simulink library "vmc"  (R2021b)
settings: Solver=VariableStepAuto  StartTime=0.0  StopTime=10.0  RelTol=1e-3
undefined symbols (not defined in the file): AVMC_ACCDeltaTqGradeGn_X_deg, AVMC_ACCDeltaTqIGain4OVRD_X_kph, AVMC_ACCDeltaTqIGain4OVRD_Y_mps2, AVMC_ACCDeltaTqIGain_X_kph, AVMC_ACCDeltaTqIGain_Y_mps2, AVMC_ACCDeltaTqPGain_X_kph, AVMC_ACCDeltaTqPGain_Y_kph, AVMC_ACCGradeofst_X_G, AVMC_ACCGradeofst_Y_pct, AVMC_ACCLoSpdTqLoLim4JP_X_kph, AVMC_ACCLoSpdTqLoLim4JP_Y_deg, AVMC_ACCLoSpdTqLowerLim_X_kph, AVMC_ACCLoSpdTqLowerLim_Y_deg, AVMC_ACCReqAccelGain_X_mps2, AVMC_ACCReqAccelGain_Y_enum, AVMC_ADSPosGFBDeltaTq_X_kph, AVMC_ADSPosGFBDeltaTq_Y_mps2, AVMC_AggressJerkPCT4AT_X_kph, AVMC_AggressJerkPCT_X_kph, AVMC_AggressLimitPCT4AT_X_kph, AVMC_AggressLimitPCT_X_kph, AVMC_DECGradeofst_X_G, AVMC_DECGradeofst_Y_pct, AVMC_DISCDeltaTqIGain_X_kph, AVMC_DISCDeltaTqIGain_Y_mps2, AVMC_DISCDeltaTqPGain_X_kph, AVMC_DISCDeltaTqPGain_Y_kph, AVMC_EPSForceSelect_X_enum, AVMC_EPSForceSelect_Y_enum, AVMC_EPSForceSelectD21_X_enum, AVMC_EPSForceSelectD21_Y_enum, AVMC_ESCRegenOut_X_kph, AVMC_ESCRegenOut_Y_Deg, AVMC_ESCRegenOutEnSpd_X_Deg, AVMC_EstPitchSlopeTs_X_kph, AVMC_GradeCompFlt_X_kph, AVMC_GyroYBandLo_X_Gps, AVMC_HoldResTq_X_kph, AVMC_ISOAccLimit_X_mps, AVMC_ISODecLimit_X_mps, AVMC_ISOJerk_X_mps, AVMC_LatESCRegenOut_X_kph, AVMC_LatESCRegenOut_Y_Deg, AVMC_LongAccDeadZone_X_kph, AVMC_LongAccFiltTsforP2_X_Gps, AVMC_MCPresBaseTq_X_bar, AVMC_MSAPedalOvrd_X_kph, AVMC_MSASpdBand_X_kph, AVMC_MSATqDownEndTq_X_kph, AVMC_MSATqDownTime_X_kph, AVMC_NegZCHoldTq_X_kph, AVMC_OPDDisSlideRate_X_Deg, AVMC_OVRD2ActSR2FCMCMD_X_mps2, AVMC_PedalTqRWhlRatio_X_Nm, AVMC_PedalTqRWhlRatio_Y_gps, AVMC_PedalTqRWhlSlipGain_X_rat, AVMC_PedalTqRWhlSlipGain_Y_kph, AVMC_PedalTqRWhSTRGGain_X_deg, AVMC_PedalTqRWhSTRGGain_Y_kph, AVMC_PosZCHoldTq_X_kph ... (+593)
libraries: hcu_lib x143, simulink x96, tqr x4, $bdroot x1, simulink_extras x1
(part 10 of 17)

== system vmc/VMC/VMC/IMU/IMU sensing result  ==
  VINP_SensingGyroX_raw16 : Inport
  VINP_SensingGyroY_raw16 : Inport  Port=2
  VINP_SensingGyroZ_raw16 : Inport  Port=3
  VINP_SensingAccX_raw16 : Inport  Port=4
  VINP_SensingAccY_raw16 : Inport  Port=5
  VINP_SensingAccZ_raw16 : Inport  Port=6
  VVMC_MemOffsetGyroX_Dps : Inport  Port=7
  VVMC_MemOffsetGyroY_Dps : Inport  Port=8
  VVMC_MemOffsetGyroZ_Dps : Inport  Port=9
  VVMC_MemOffsetAccX_G : Inport  Port=10
  VVMC_MemOffsetAccY_G : Inport  Port=11
  VVMC_MemOffsetAccZ_G : Inport  Port=12
  task_time_s : Inport  Port=13
  ACCEL_FS_SEL = 001 SENSITIVITY = 2000 LSB/g : Constant  Value=KVMC_AccFSSlect_enum
  Add{1..5,8} (6 alike) : Sum
  Cast To Single{1,4,7,10,14,17} (6 alike) : DataTypeConversion  OutDataTypeStr=single
  Cast To Single{2..3,5..6,8..9,11..13,15..16,18} (12 alike) : DataTypeConversion  OutDataTypeStr=uint8
  Constant{1..2,4,6} (4 alike) : Constant  Value=MINUSONE_FLOAT
  Constant{10,13,16,19..20,25} (6 alike) : Constant  Value=ZERO_FLOAT
  Constant{11,14,17,21..22,26,29..34} (12 alike) : Constant  Value=ONE_INT
  Constant12 : Constant  Value=KVMC_IMUGyroYRollAveLevel_enum
  Constant15 : Constant  Value=KVMC_IMUGyroZRollAveLevel_enum
  Constant18 : Constant  Value=KVMC_IMUAccXRollAveLevel_enum
  Constant23 : Constant  Value=KVMC_IMUGxFilter_raw32
  Constant24 : Constant  Value=KVMC_IMUAccYRollAveLevel_enum
  Constant27 : Constant  Value=KVMC_IMUGyroXRollAveLevel_enum
  Constant28 : Constant  Value=KVMC_IMUAccZRollAveLevel_enum
  Constant3 : Constant  Value=KVMC_IMURxFilter_raw32
  Constant5 : Constant  Value=KVMC_IMURzFilter_raw32
  Constant7 : Constant  Value=KVMC_IMUGzFilter_raw32
  Constant8 : Constant  Value=KVMC_IMUGyFilter_raw32
  Constant9 : Constant  Value=KVMC_IMURyFilter_raw32
  Data Type Conversion : DataTypeConversion  OutDataTypeStr=uint16
  Data Type Conversion{1..6} (6 alike) : DataTypeConversion  OutDataTypeStr=single
  Data Type Conversion7 : DataTypeConversion  OutDataTypeStr=uint16
  Divide{,1..9} (10 alike) : Product  Inputs=**
  FirstOrderFilter{1..6} (6 alike) : hcu_lib/Basic_Blocks/FirstOrderFilter
  GYRO_FS_SEL = 0001 SENSITIVITY = 50 LSB/dps : Constant  Value=KVMC_GyroFSSlect_enum
  Math Function{,1..5} (6 alike) : Math  Operator=reciprocal  SaturateOnIntegerOverflow=on
  Min{1..6} (6 alike) : MinMax  Function=max  Inputs=2
  Plus{,1..5} (6 alike) : Sum  Inputs=+-
  RollingAverage : Stateflow chart  TreatAsAtomicUnit=on
  RollingAverage1 : Stateflow chart  TreatAsAtomicUnit=on
  RollingAverage2 : Stateflow chart  TreatAsAtomicUnit=on
  RollingAverage3 : Stateflow chart  TreatAsAtomicUnit=on
  RollingAverage4 : Stateflow chart  TreatAsAtomicUnit=on
  RollingAverage5 : Stateflow chart  TreatAsAtomicUnit=on
  VVMC_CalibratedGyroX_Dps : Outport
  VVMC_CalibratedGyroY_Dps : Outport  Port=2
  VVMC_CalibratedGyroZ_Dps : Outport  Port=3
  VVMC_CalibratedAccX_G : Outport  Port=4
  VVMC_CalibratedAccY_G : Outport  Port=5
  VVMC_CalibratedAccZ_G : Outport  Port=6
  VVMC_CalibratedAccXAftRA_G : Outport  Port=7
  wires:
  [VVMC_CalibratedAccXAftRA_G] -> VVMC_CalibratedAccXAftRA_G/1
  Min6/1 -> RollingAverage5/1(KVMC_RollAveLevel_enum)
  Constant34/1 -> Min6/2
  Min5/1 -> RollingAverage4/1(KVMC_RollAveLevel_enum)
  Constant33/1 -> Min5/2
  Min4/1 -> RollingAverage3/1(KVMC_RollAveLevel_enum)
  Constant32/1 -> Min4/2
  Min2/1 -> RollingAverage2/1(KVMC_RollAveLevel_enum)
  Constant31/1 -> Min2/2
  Min1/1 -> RollingAverage1/1(KVMC_RollAveLevel_enum)
  Constant30/1 -> Min1/2
  Min3/1 -> RollingAverage/1(KVMC_RollAveLevel_enum)
  Constant29/1 -> Min3/2
  [VVMC_CalibratedAccZ_G] -> VVMC_CalibratedAccZ_G/1
  [VVMC_CalibratedAccY_G] -> VVMC_CalibratedAccY_G/1
  [VVMC_CalibratedAccX_G] -> VVMC_CalibratedAccX_G/1
  [VVMC_CalibratedGyroZ_Dps] -> VVMC_CalibratedGyroZ_Dps/1
  [VVMC_CalibratedGyroY_Dps] -> VVMC_CalibratedGyroY_Dps/1
  [VVMC_CalibratedGyroX_Dps] -> VVMC_CalibratedGyroX_Dps/1
  RollingAverage5/1(VVMC_RollAve_raw32) -> FirstOrderFilter3/1
  Constant25/1 -> Cast To Single17/1
  Constant28/1 -> Cast To Single16/1
  Cast To Single18/1 -> RollingAverage5/3(ONE_INT)
  Cast To Single16/1 -> Min6/1
  Cast To Single17/1 -> RollingAverage5/2(ZERO_FLOAT)
  Constant26/1 -> Cast To Single18/1
  RollingAverage4/1(VVMC_RollAve_raw32) -> FirstOrderFilter4/1
  Constant22/1 -> Cast To Single15/1
  Cast To Single14/1 -> RollingAverage4/2(ZERO_FLOAT)
  Cast To Single13/1 -> Min5/1
  Cast To Single15/1 -> RollingAverage4/3(ONE_INT)
  Constant24/1 -> Cast To Single13/1
  Constant19/1 -> Cast To Single14/1
  RollingAverage3/1(VVMC_RollAve_raw32) -> [VVMC_CalibratedAccXAftRA_G], FirstOrderFilter6/1  "VVMC_CalibratedAccXAftRA_G"
  Constant16/1 -> Cast To Single7/1
  Constant18/1 -> Cast To Single11/1
  Cast To Single8/1 -> RollingAverage3/3(ONE_INT)
  Cast To Single11/1 -> Min4/1
  Cast To Single7/1 -> RollingAverage3/2(ZERO_FLOAT)
  Constant17/1 -> Cast To Single8/1
  RollingAverage2/1(VVMC_RollAve_raw32) -> FirstOrderFilter2/1
  Cast To Single5/1 -> RollingAverage2/3(ONE_INT)
  Cast To Single4/1 -> RollingAverage2/2(ZERO_FLOAT)
  Cast To Single6/1 -> Min2/1
  Constant14/1 -> Cast To Single5/1
  Constant15/1 -> Cast To Single6/1
  Constant13/1 -> Cast To Single4/1
  RollingAverage1/1(VVMC_RollAve_raw32) -> FirstOrderFilter5/1
  Constant10/1 -> Cast To Single1/1
  Constant12/1 -> Cast To Single3/1
  Cast To Single2/1 -> RollingAverage1/3(ONE_INT)
  Cast To Single3/1 -> Min1/1
  Cast To Single1/1 -> RollingAverage1/2(ZERO_FLOAT)
  Constant11/1 -> Cast To Single2/1
  RollingAverage/1(VVMC_RollAve_raw32) -> FirstOrderFilter1/1
  Constant21/1 -> Cast To Single12/1
  Cast To Single10/1 -> RollingAverage/2(ZERO_FLOAT)
  Cast To Single9/1 -> Min3/1
  Cast To Single12/1 -> RollingAverage/3(ONE_INT)
  Constant27/1 -> Cast To Single9/1
  Constant20/1 -> Cast To Single10/1
  Plus1/1 -> RollingAverage1/4(VINP_INPData_raw32)
  Add5/1 -> FirstOrderFilter5/3
  Constant9/1 -> Add5/2
  [task_time_s] -> FirstOrderFilter5/2, Add5/1
  Plus4/1 -> RollingAverage4/4(VINP_INPData_raw32)
  [task_time_s] -> Add4/1, FirstOrderFilter4/2
  Constant8/1 -> Add4/2
  Add4/1 -> FirstOrderFilter4/3
  Plus5/1 -> Divide9/1
  [task_time_s] -> Add3/1, FirstOrderFilter3/2
  Constant7/1 -> Add3/2
  Add3/1 -> FirstOrderFilter3/3
  Constant6/1 -> Divide9/2
  Divide9/1 -> RollingAverage5/4(VINP_INPData_raw32)
  Plus2/1 -> Divide8/1
  Divide8/1 -> RollingAverage2/4(VINP_INPData_raw32)
  Constant4/1 -> Divide8/2
  Add2/1 -> FirstOrderFilter2/3
  Constant5/1 -> Add2/2
  [task_time_s] -> FirstOrderFilter2/2, Add2/1
  Plus/1 -> Divide7/1
  [task_time_s] -> Add1/1, FirstOrderFilter1/2
  Constant3/1 -> Add1/2
  Add1/1 -> FirstOrderFilter1/3
  Constant2/1 -> Divide7/2
  Divide7/1 -> RollingAverage/4(VINP_INPData_raw32)
  Divide6/1 -> RollingAverage3/4(VINP_INPData_raw32)
  Constant1/1 -> Divide6/2
  Add8/1 -> FirstOrderFilter6/3
  Constant23/1 -> Add8/2
  Plus3/1 -> Divide6/1
  [task_time_s] -> FirstOrderFilter6/2, Add8/1
  task_time_s/1 -> [task_time_s]
  Data Type Conversion6/1 -> Math Function5/1
  [VVMC_AccFSSlect_enum] -> Data Type Conversion6/1
  Data Type Conversion5/1 -> Math Function4/1
  Data Type Conversion4/1 -> Math Function3/1
  [VVMC_AccFSSlect_enum] -> Data Type Conversion4/1
  Data Type Conversion3/1 -> Math Function2/1
  Data Type Conversion2/1 -> Math Function1/1
  Data Type Conversion1/1 -> Math Function/1
  Math Function5/1 -> Divide5/2
  Math Function4/1 -> Divide4/2
  Math Function3/1 -> Divide3/2
  Math Function2/1 -> Divide2/2
  Math Function1/1 -> Divide1/2
  Math Function/1 -> Divide/2
  FirstOrderFilter3/1 -> [VVMC_CalibratedAccZ_G]  "VVMC_CalibratedAccZ_G"
  FirstOrderFilter4/1 -> [VVMC_CalibratedAccY_G]  "VVMC_CalibratedAccY_G"
  FirstOrderFilter6/1 -> [VVMC_CalibratedAccX_G]  "VVMC_CalibratedAccX_G"
  FirstOrderFilter2/1 -> [VVMC_CalibratedGyroZ_Dps]  "VVMC_CalibratedGyroZ_Dps"
  FirstOrderFilter5/1 -> [VVMC_CalibratedGyroY_Dps]  "VVMC_CalibratedGyroY_Dps"
  FirstOrderFilter1/1 -> [VVMC_CalibratedGyroX_Dps]  "VVMC_CalibratedGyroX_Dps"
  [VVMC_MemOffsetAccZ_G] -> Plus5/2
  [VVMC_SensingAccZ_G] -> Plus5/1
  [VVMC_MemOffsetAccY_G] -> Plus4/2
  [VVMC_SensingAccY_G] -> Plus4/1
  [VVMC_MemOffsetAccX_G] -> Plus3/2
  [VVMC_SensingAccX_G] -> Plus3/1
  [VVMC_MemOffsetGyroZ_Dps] -> Plus2/2
  [VVMC_SensingGyroZ_Dps] -> Plus2/1
  [VVMC_MemOffsetGyroY_Dps] -> Plus1/2
  [VVMC_SensingGyroY_Dps] -> Plus1/1
  [VVMC_MemOffsetGyroX_Dps] -> Plus/2
  [VVMC_SensingGyroX_Dps] -> Plus/1
  Divide/1 -> [VVMC_SensingGyroX_Dps]  "VVMC_SensingGyroX_Dps"
  Divide5/1 -> [VVMC_SensingAccZ_G]  "VVMC_SensingAccZ_G"
  VINP_SensingAccZ_raw16/1 -> [VINP_SensingAccZ_raw16]
  VINP_SensingAccY_raw16/1 -> [VINP_SensingAccY_raw16]
  VINP_SensingAccX_raw16/1 -> [VINP_SensingAccX_raw16]
  VINP_SensingGyroZ_raw16/1 -> [VINP_SensingGyroZ_raw16]
  VINP_SensingGyroY_raw16/1 -> [VINP_SensingGyroY_raw16]
  VINP_SensingGyroX_raw16/1 -> [VINP_SensingGyroX_raw16]
  VVMC_MemOffsetAccX_G/1 -> [VVMC_MemOffsetAccX_G]
  VVMC_MemOffsetGyroZ_Dps/1 -> [VVMC_MemOffsetGyroZ_Dps]
  VVMC_MemOffsetAccZ_G/1 -> [VVMC_MemOffsetAccZ_G]
  VVMC_MemOffsetAccY_G/1 -> [VVMC_MemOffsetAccY_G]
  VVMC_MemOffsetGyroX_Dps/1 -> [VVMC_MemOffsetGyroX_Dps]
  VVMC_MemOffsetGyroY_Dps/1 -> [VVMC_MemOffsetGyroY_Dps]
  [VINP_SensingGyroX_raw16] -> Divide/1
  [VVMC_GyroFSSlect_enum] -> Data Type Conversion1/1
  GYRO_FS_SEL = 0001 SENSITIVITY = 50 LSB/dps/1 -> Data Type Conversion/1
  Data Type Conversion/1 -> [VVMC_GyroFSSlect_enum]  "VVMC_GyroFSSlect_enum"
  [VVMC_GyroFSSlect_enum] -> Data Type Conversion2/1
  [VINP_SensingGyroY_raw16] -> Divide1/1
  [VINP_SensingGyroZ_raw16] -> Divide2/1
  [VVMC_GyroFSSlect_enum] -> Data Type Conversion3/1
  [VINP_SensingAccX_raw16] -> Divide3/1
  [VINP_SensingAccY_raw16] -> Divide4/1
  [VVMC_AccFSSlect_enum] -> Data Type Conversion5/1
  [VINP_SensingAccZ_raw16] -> Divide5/1
  Data Type Conversion7/1 -> [VVMC_AccFSSlect_enum]  "VVMC_AccFSSlect_enum"
  ACCEL_FS_SEL = 001 SENSITIVITY = 2000 LSB/g/1 -> Data Type Conversion7/1
  Divide1/1 -> [VVMC_SensingGyroY_Dps]  "VVMC_SensingGyroY_Dps"
  Divide2/1 -> [VVMC_SensingGyroZ_Dps]  "VVMC_SensingGyroZ_Dps"
  Divide3/1 -> [VVMC_SensingAccX_G]  "VVMC_SensingAccX_G"
  Divide4/1 -> [VVMC_SensingAccY_G]  "VVMC_SensingAccY_G"

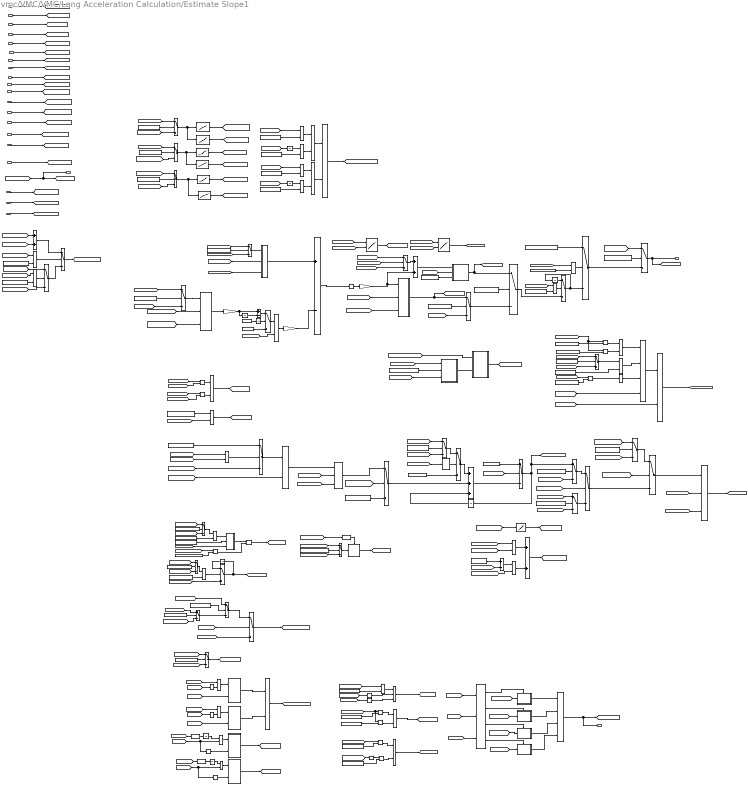
== system vmc/VMC/VMC/Long Acceleration Calculation/Estimate Slope1 ==
  VINP_LongAccel_Gps : Inport
  VINP_VehSpeed_kph : Inport  Port=2
  VINP_GRADE_deg : Inport  Port=3
  VVMC_CalibratedGyroY_Dps : Inport  Port=4
  VVMC_CalibratedAccX_G : Inport  Port=5
  VVMC_CalibratedAccY_G : Inport  Port=6
  VVMC_CalibratedAccZ_G : Inport  Port=7
  C_TASK_10MS_S : Inport  Port=8
  VDHP_ActAPSPosn_pct : Inport  Port=9
  VTQD_GearActualPosn_enum : Inport  Port=10
  VTQD_PreLoadPreEn_flg : Inport  Port=11
  VINP_BrkPedalPos_pct : Inport  Port=12
  VTQD_VehActSpd_kph : Inport  Port=13
  VTQD_RegenMode_enum : Inport  Port=14
  VINP_DIDGetDynoMode_flg : Inport  Port=15
  VVMC_HoldEstSlope_deg : Inport  Port=16
  VVMC_InitEstSlope_Deg : Inport  Port=17
  VTQR_RrTMTqReq_Nm : Inport  Port=18
  VTQR_FrTMTqReq_Nm : Inport  Port=19
  VPMM_DrivetrainSelect_enum : Inport  Port=20
  AND{,2..12} (12 alike) : Logic  AllPortsSameDT=off  OutDataTypeStr=boolean
  AND1 : Logic  Inputs=4  AllPortsSameDT=off  OutDataTypeStr=boolean
  AND13 : Logic  Inputs=3  AllPortsSameDT=off  OutDataTypeStr=boolean
  Abs : Abs
  Add : Sum
  Add1 : Sum  Inputs=+-
  Add2 : Sum  Inputs=+++
  Add3 : Sum
  Add5 : Sum
  Asin1 : Trigonometry  Operator=asin
  Constant : Constant  Value=KVMC_EstSlopeVehSourceSW_flg
  Constant1 : Constant  Value=KVMC_VehRunSlope_flg
  Constant{10,12,25,31,53} (5 alike) : Constant  Value=ZERO_FLOAT
  Constant11 : Constant  Value=KVMC_PitchVehThres_kph
  Constant13 : Constant  Value=KVMC_VehStopAPSThresLo_pct
  Constant14 : Constant  Value=KVMC_DIDGetDynoModeSW_flg
  Constant{15,36,50..51} (4 alike) : Constant  Value=KVMC_SlopeCalSource_flg
  Constant16 : Constant  Value=KVMC_PitchBPSThres_pct
  Constant17 : Constant  Value=ENUM_GEARSHIFTCMD_D
  Constant18 : Constant  Value=ENUM_GEARSHIFTCMD_R
  Constant19 : Constant  Value=ENUM_GEARSHIFTCMD_R
  Constant2 : Constant  Value=ENUM_DRIVETRAIN_AWD
  Constant20 : Constant  Value=KVMC_GyroBandSource_flg
  Constant21 : Constant  Value=ENUM_GEARSHIFTCMD_D
  Constant22 : Constant  Value=KVMC_GradedelayTimer_s
  Constant23 : Constant  Value=KVMC_VehStopSource_flg
  Constant24 : Constant  Value=KVMC_GradedelaytestSW_flg
  Constant26 : Constant  Value=KVMC_PitchGradeReset_flg
  Constant27 : Constant  Value=KVMC_PitchGradeStopSource_flg
  Constant29 : Constant  Value=KVMC_PitchGradeStopSource_flg
  Constant3 : Constant  Value=ENUM_DRIVETRAIN_RWD
  Constant30 : Constant  Value=KVMC_VehStopThres_kph
  Constant32 : Constant  Value=KVMC_VehStopDelay_s
  Constant33 : Constant  Value=KVMC_VehStopThresLo_kph
  Constant34 : Constant  Value=KVMC_VehStopThresHi_kph
  Constant35 : Constant  Value=KVMC_VehStopThresHi_kph
  Constant38 : Constant  Value=KVMC_VehStopThresLo_kph
  Constant39 : Constant  Value=KVMC_EstSlopeVehSourceSW_flg
  Constant4 : Constant  Value=KVMC_VehStopTqThres_Nm
  Constant42 : Constant  Value=KVMC_EstSlopeSW_flg
  Constant47 : Constant  Value=KVMC_CalEstSlopeOfst_c
  Constant48 : Constant  Value=KVMC_CalEstSlopeOfstSW_flg
  Constant49 : Constant  Value=KVMC_FreezeStopGrade_kph
  Constant5 : Constant  Value=ONE_FLOAT
  Constant52 : Constant  Value=KVMC_EstSlopeLongGSW_flg
  Constant54 : Constant  Value=KVMC_PitchAccGup_mps2
  Constant55 : Constant  Value=KVMC_PitchAccGlow_mps2
  Constant56 : Constant  Value=KVMC_EstSlopeVehSourceSW_flg
  Constant57 : Constant  Value=KVMC_StoploopGradeSource_flg
  Constant6 : Constant  Value=KVMC_PitchGradeL2HSource_flg
  Constant60 : Constant  Tag=struct('comment',struct('text','','placement',1),'output',struct('width',1,'name','$S_$B','unit','','type','Int16','offset',0,'max',NaN,'min',NaN,'freeze',1,'lsb',1,'arb',0,'class','default','address','','description','','value','2','tolerance',1,'show',0),'date',731450.690075)  Value=TRUE
  Constant7 : Constant  Value=KVMC_VehStopSource_flg
  Constant8 : Constant  Tag=struct('comment',struct('text','','placement',1),'output',struct('width',1,'name','$S_$B','unit','','type','Int16','offset',0,'max',NaN,'min',NaN,'freeze',1,'lsb',1,'arb',0,'class','default','address','','description','','value','0','tolerance',1,'show',0),'date',731450.689904282)  Value=ZERO_FLOAT  OutDataTypeStr=single
  Constant9 : Constant  Value=KVMC_SlopeSourceTs_flg
  DelayEnable : Subsystem  mask(DelayEnable){}
      mask help: Delay enable funcion.
  DelayEnable4 : Subsystem  mask(DelayEnable){}
      mask help: Delay enable funcion.
  Detect Decrease{,1..3} (4 alike) : simulink/Logic and Bit Operations/Detect Decrease  vinit=0.0  OutDataTypeStr=boolean
  Equal{,1..5} (6 alike) : RelationalOperator  Operator===  OutDataTypeStr=boolean  RndMeth=Simplest
  FirstOrderFilter3 : Subsystem  RTWFileName=HCU_LIB  mask(FirstOrderFilter){}
      mask help: First order Filter.
      settings: RTWFileNameOpts=User specified
  FirstOrderFilter4 : Subsystem  RTWFileName=HCU_LIB  mask(FirstOrderFilter){}
      mask help: First order Filter.
      settings: RTWFileNameOpts=User specified
  FirstOrderFilter5 : Subsystem  RTWFileName=HCU_LIB  mask(FirstOrderFilter){}
      mask help: First order Filter.
      settings: RTWFileNameOpts=User specified
  FirstOrderFilter6 : Subsystem  RTWFileName=HCU_LIB  mask(FirstOrderFilter){}
      mask help: First order Filter.
      settings: RTWFileNameOpts=User specified
  FirstOrderFilter7 : Subsystem  RTWFileName=HCU_LIB  mask(FirstOrderFilter){}
      mask help: First order Filter.
      settings: RTWFileNameOpts=User specified
  FirstOrderFilter8 : Subsystem  RTWFileName=HCU_LIB  mask(FirstOrderFilter){}
      mask help: First order Filter.
      settings: RTWFileNameOpts=User specified
  Gain : Gain  Gain=KPH2MPS
  Gain1 : Gain  Gain=1/GRAVITY_G
  Gain5 : Gain  Gain=RAD2DEG
  GreaterThan : RelationalOperator  Operator=<  OutDataTypeStr=boolean  RndMeth=Simplest
  GreaterThan2 : RelationalOperator  OutDataTypeStr=boolean  RndMeth=Simplest
  GreaterThan3 : RelationalOperator  Operator=>  OutDataTypeStr=boolean  RndMeth=Simplest
  GreaterThan4 : RelationalOperator  Operator=>  OutDataTypeStr=boolean  RndMeth=Simplest
  GreaterThan5 : RelationalOperator  Operator=>  OutDataTypeStr=boolean  RndMeth=Simplest
  If : If  NumInputs=3  IfExpression=u1 ~= 0  ElseIfExpressions=u2 ~= 0, u3~=0
  If Action Subsystem : Subsystem  TreatAsAtomicUnit=on
  If Action Subsystem1 : Subsystem  TreatAsAtomicUnit=on
  If Action Subsystem2 : Subsystem  TreatAsAtomicUnit=on
  If Action Subsystem3 : Subsystem  TreatAsAtomicUnit=on
  Less Than : RelationalOperator  Operator=>  OutDataTypeStr=boolean  RndMeth=Simplest
  Less Than{1..2,5..8} (6 alike) : RelationalOperator  Operator=<  OutDataTypeStr=boolean  RndMeth=Simplest
  Less Than3 : RelationalOperator  OutDataTypeStr=boolean  RndMeth=Simplest
  Less Than4 : RelationalOperator  Operator=<=  OutDataTypeStr=boolean  RndMeth=Simplest
  MVMC_ACCGradeofst_Deg : Lookup_n-D  BreakpointsForDimension1=AVMC_ACCGradeofst_Y_pct  BreakpointsForDimension2=AVMC_ACCGradeofst_X_G  Table=MVMC_ACCGradeofst_Z_Deg  InternalRulePriority=Speed  RndMeth=Simplest  InputSameDT=on
      settings: InputPortMap=u0,u1
  MVMC_CalEstSlopeTs_Y_c : Lookup_n-D  NumberOfTableDimensions=1  BreakpointsForDimension1=AVMC_EstPitchSlopeTs_X_kph  Table=MVMC_CalEstSlopeTs_Y_c  InternalRulePriority=Speed  RndMeth=Simplest  InputSameDT=on
  MVMC_CalibratedGyroYDevTs_Y_c : Lookup_n-D  NumberOfTableDimensions=1  BreakpointsForDimension1=AVMC_EstPitchSlopeTs_X_kph  Table=MVMC_CalibratedGyroYDevTs_Y_c  InternalRulePriority=Speed  RndMeth=Simplest  InputSameDT=on
  MVMC_DECGradeofst_Deg : Lookup_n-D  BreakpointsForDimension1=AVMC_DECGradeofst_Y_pct  BreakpointsForDimension2=AVMC_DECGradeofst_X_G  Table=MVMC_DECGradeofst_Z_Deg  InternalRulePriority=Speed  RndMeth=Simplest  InputSameDT=on
      settings: InputPortMap=u0,u1
  MVMC_EstPitchSlopeTs_Y_c : Lookup_n-D  NumberOfTableDimensions=1  BreakpointsForDimension1=AVMC_EstPitchSlopeTs_X_kph  Table=MVMC_EstPitchSlopeTs_Y_c  InternalRulePriority=Speed  RndMeth=Simplest  InputSameDT=on
  MVMC_GradeCompFlt_Y_c : Lookup_n-D  NumberOfTableDimensions=1  BreakpointsForDimension1=AVMC_GradeCompFlt_X_kph  Table=MVMC_GradeCompFlt_Y_c  InternalRulePriority=Speed  RndMeth=Simplest  InputSameDT=on
  MVMC_GyroYBandHi_Y_Dps : Lookup_n-D  NumberOfTableDimensions=1  BreakpointsForDimension1=AVMC_GyroYBandLo_X_Gps  Table=MVMC_GyroYBandHi_Y_Dps  InternalRulePriority=Speed  RndMeth=Simplest  InputSameDT=on
  MVMC_GyroYBandLo_Y_Dps : Lookup_n-D  NumberOfTableDimensions=1  BreakpointsForDimension1=AVMC_GyroYBandLo_X_Gps  Table=MVMC_GyroYBandLo_Y_Dps  InternalRulePriority=Speed  RndMeth=Simplest  InputSameDT=on
  MVMC_VehspdTs_Y_c : Lookup_n-D  NumberOfTableDimensions=1  BreakpointsForDimension1=AVMC_EstPitchSlopeTs_X_kph  Table=MVMC_VehspdTs_Y_c  InternalRulePriority=Speed  RndMeth=Simplest  InputSameDT=on
  Merge : Merge  Inputs=4
  NOT{,1..4,7..8} (7 alike) : Logic  Operator=NOT  AllPortsSameDT=off  OutDataTypeStr=boolean
  OR{,3,5..7} (5 alike) : Logic  Operator=OR  AllPortsSameDT=off  OutDataTypeStr=boolean
  OR1 : Logic  AllPortsSameDT=off  OutDataTypeStr=boolean
  Product : Product
  Product1 : Product
  Product2 : Product
  Product4 : Product  Tag=struct('comment',struct('text','','placement',1),'logdata',struct('maxnumvals',inf,'plotchannels',[],'stepsize',0,'downsampling',1,'loggingmode',3,'channels',1),'output',struct('width',1,'name','$S_$B','unit','','type','Int32Bin15','offset',0,'max',65535,'min',-65536,'freeze',1,'lsb',2^-15,'arb',0,'class','default','address','','description','','autoscalingmode',1,'lowerheadroom',1,'upperheadroom',1,'headroomunit','bit','checkmin',0,'checkmax',0,'show',0),'inputs','*/','exceptionhandling',1,'date',731458.438505301)  Inputs=*/  InputSameDT=on  RndMeth=Zero  SaturateOnIntegerOverflow=on  OutDataTypeStr=Inherit: Same as first input
  SR_Latch : Subsystem  mask(SR_Latch){}
      mask help: SR latch function.
  SR_Latch1 : Subsystem  mask(SR_Latch){}
      mask help: SR latch function.
  SR_Latch2 : Subsystem  mask(SR_Latch){}
      mask help: SR latch function.
  SR_Latch3 : Subsystem  mask(SR_Latch){}
      mask help: SR latch function.
  SR_Latch6 : Subsystem  mask(SR_Latch){}
      mask help: SR latch function.
  Subtract : Sum  Inputs=+-
  Sum1 : Sum  Tag=struct('comment',struct('text','','placement',1),'logdata',struct('maxnumvals',inf,'plotchannels',[],'stepsize',0,'downsampling',1,'loggingmode',3,'channels',1),'output',struct('width',1,'name','$S_$B','unit','','type','Int32Bin15','offset',0,'max',65535,'min',-65536,'freeze',1,'lsb',2^-15,'arb',0,'class','default','address','','description','','autoscalingmode',1,'lowerheadroom',1,'upperheadroom',1,'headroomunit','bit','checkmin',0,'checkmax',0,'show',0),'inputs','+-','date',731450.688943275)  Inputs=+-  InputSameDT=on  SaturateOnIntegerOverflow=on  OutDataTypeStr=Inherit: Same as first input
  Switch{,1..3,8,12,14..23,25..28,30..31,33} (23 alike) : Switch  Criteria=u2 > Threshold
  Switch{4..7,9..11,32} (8 alike) : Switch  Criteria=u2 ~= 0
  Switch13 : Switch
  Switch35 : Switch  Tag=struct('comment',struct('text','','placement',1),'logdata',struct('maxnumvals',inf,'plotchannels',[],'stepsize',0,'downsampling',1,'loggingmode',3,'channels',1),'output',struct('width',1,'name','$S_$B','unit','','type','Int32Bin15','offset',0,'max',65535,'min',-65536,'freeze',1,'lsb',2^-15,'arb',0,'class','default','address','','description','','autoscalingmode',1,'lowerheadroom',1,'upperheadroom',1,'headroomunit','bit','checkmin',0,'checkmax',0,'show',0),'threshold',struct('width',1,'name','$S_$B_threshold','unit','','type','Int16','offset',0,'max',NaN,'min',NaN,'freeze',1,'lsb',1,'arb',0,'class','default','address','','description','','value','1','scalar',0),'date',731458.438569977)  Criteria=u2 > Threshold  SaturateOnIntegerOverflow=on  InputSameDT=on
  Triggered Subsystem : Subsystem  TreatAsAtomicUnit=on
  Unit Delay{,1..5,8} (7 alike) : UnitDelay  SampleTime=-1  HasFrameUpgradeWarning=on
  UnitDelay3 : UnitDelay  Tag=struct('comment',struct('text','','placement',1),'logdata',struct('maxnumvals',inf,'plotchannels',[],'stepsize',0,'downsampling',1,'loggingmode',3,'channels',1),'output',struct('width',1,'name','$S_$B','unit','','type','Int32Bin15','offset',0,'max',65535,'min',-65536,'freeze',1,'lsb',2^-15,'arb',0,'class','default','address','','description','','autoscalingmode',1,'lowerheadroom',1,'upperheadroom',1,'headroomunit','bit','checkmin',0,'checkmax',0,'show',0,'initial','0'),'state',0,'dt','-1','date',731450.687911019)  SampleTime=-1  HasFrameUpgradeWarning=on
  UnitDelay4 : UnitDelay  Tag=struct('comment',struct('text','','placement',1),'logdata',struct('maxnumvals',inf,'plotchannels',[],'stepsize',0,'downsampling',1,'loggingmode',3,'channels',1),'output',struct('width',1,'name','$S_$B','unit','','type','UInt8','offset',0,'max',255,'min',0,'freeze',1,'lsb',1,'arb',0,'class','default','address','','description','','autoscalingmode',1,'lowerheadroom',1,'upperheadroom',1,'headroomunit','bit','checkmin',0,'checkmax',0,'show',0,'initial','0'),'state',0,'dt','-1','date',731450.690382801)  InitialCondition=FALSE  SampleTime=-1  StateName=first_pass  HasFrameUpgradeWarning=on
  VVMC_EstSlopeCalBase_Deg : Outport
  VVMC_IMUEstSlope_Deg1 : Outport  Port=2
  VVMC_FinalSlop_deg : Outport  Port=3
  wires:
  C_TASK_10MS_S/1 -> [task_time_s]
  [VINP_GRADE_deg] -> Switch1/3
  [VINP_LongAccel_Gps] -> Switch3/3
  VVMC_CalibratedAccZ_G/1 -> [VVMC_CalibratedAccZ_G]
  VVMC_CalibratedAccY_G/1 -> [VVMC_CalibratedAccY_G]
  Switch33/1 -> Switch26/1
  [VVMC_PitchIntegGradeMen_deg] -> Switch33/1
  Constant57/1 -> Switch33/2
  [VVMC_PitchIntegGradeMen_deg] -> Switch26/3
  [VVMC_EstSlopeCalBase_Deg] -> Switch/1
  [VVMC_DECGradeofst_Deg] -> Switch22/3
  FirstOrderFilter4/1(out) -> Gain/1
  SR_Latch6/1(latched) -> [VVMC_GradeShiftDelay_flg]  "VVMC_GradeShiftDelay_flg"
  [VVMC_EstSlopeCalBase_Deg] -> Switch30/1
  [VVMC_StopGrade_deg] -> If Action Subsystem2/1(In1)
  Constant17/1 -> Equal2/2
  Switch30/1 -> Switch13/1
  Switch4/1 -> FirstOrderFilter4/1(in)
  [VINP_BrkPedalPos_pct] -> MVMC_DECGradeofst_Deg/1
  [VVMC_EstSlopeCalBase_Deg] -> Switch31/1
  GreaterThan3/1 -> NOT/1
  MVMC_GyroYBandHi_Y_Dps/1 -> [VVMC_GyroYBandHigh_Dps]  "VVMC_GyroYBandHigh_Dps"
  AND10/1 -> SR_Latch2/1(set)
  [VVMC_GyroYBand_flg] -> OR3/1
  [VTQD_VehActSpd_kph] -> Switch4/1
  Switch2/1 -> Switch31/3
  [task_time_s] -> FirstOrderFilter4/2(Tc)
  DelayEnable/1(set) -> AND9/1
  [VVMC_EstSlopeCalBase_Deg] -> Switch28/1
  FirstOrderFilter5/1(out) -> Switch1/1, [VVMC_CalEstSlope1_Deg]  "VVMC_CalEstSlope1_Deg"
  [task_time_s] -> FirstOrderFilter6/2(Tc)
  [VTQD_PreLoadPreEn_flg] -> DelayEnable4/1(trigger)
  [VDHP_ActAPSPosn_pct] -> MVMC_ACCGradeofst_Deg/1
  [VVMC_CalibratedGyroY_Dps] -> GreaterThan4/1
  Constant26/1 -> OR7/1
  [VVMC_ACCGradeofst_Deg] -> Switch22/1
  [VTQD_VehActSpd_kph] -> Switch20/1
  Less Than1/1 -> OR1/2
  [VVMC_GradeReset_flg] -> Switch12/2
  [VVMC_CalibratedAccX_G] -> MVMC_DECGradeofst_Deg/2
  Switch22/1 -> Add5/1
  [VVMC_Vehfullstop_flg] -> Switch26/2
  FirstOrderFilter8/1(out) -> [VVMC_CalEstSlopeOfstA_Deg], Switch23/1  "VVMC_CalEstSlopeOfstA_Deg"
  MVMC_CalibratedGyroYDevTs_Y_c/1 -> [VVMC_CalibratedGyroYDevTs_c]  "VVMC_CalibratedGyroYDevTs_c"
  [VVMC_CalibratedAccX_G] -> Switch10/1
  Merge/1 -> [VVMC_FinalSlop_deg], VVMC_FinalSlop_deg/1  "VVMC_FinalSlop_deg"
  Switch9/1 -> Product/1
  [VVMC_HoldEstSlope_deg] -> Switch28/3
  [VVMC_GyroYBandLow_Dps] -> GreaterThan4/2
  Switch15/1 -> MVMC_VehspdTs_Y_c/1, MVMC_CalEstSlopeTs_Y_c/1
  Constant39/1 -> Switch32/2
  If Action Subsystem2/1(Out1) -> Merge/3
  Constant32/1 -> DelayEnable/2(T_delay)
  Constant53/1 -> Switch2/1
  [VINP_VehSpeed_kph] -> Switch20/3
  Constant47/1 -> FirstOrderFilter8/3(Ts)
  Add5/1 -> FirstOrderFilter8/1(in)  "VVMC_CalEstSlopeOfstB_Deg"
  Constant21/1 -> Equal4/2
  Constant9/1 -> Switch15/2
  Switch16/1 -> Triggered Subsystem/1(In1)
  [task_time_s] -> FirstOrderFilter3/2(Tc)
  [VTQD_VehActSpd_kph] -> Switch15/3
  Constant54/1 -> GreaterThan/2
  [VVMC_CalibratedAccX_G] -> Switch15/1
  If/1 -> If Action Subsystem/Action
  MVMC_DECGradeofst_Deg/1 -> [VVMC_DECGradeofst_Deg]  "VVMC_DECGradeofst_Deg"
  [VVMC_GyroYBandHigh_Dps] -> Less Than1/2
  MVMC_ACCGradeofst_Deg/1 -> [VVMC_ACCGradeofst_Deg]  "VVMC_ACCGradeofst_Deg"
  Constant34/1 -> Less Than4/2
  Gain5/1 -> FirstOrderFilter5/1(in), Add5/2  "VVMC_CalEstSlopeBefore_Deg"
  OR1/1 -> [VVMC_GyroYBand_flg]  "VVMC_GyroYBand_flg"
  [VVMC_GradeReset_flg] -> OR3/2
  Less Than7/1 -> Switch25/2
  OR3/1 -> Switch9/2
  [VVMC_VehspdLo_flg] -> SR_Latch1/2(reset)
  AND7/1 -> Switch8/2
  VVMC_CalibratedAccX_G/1 -> [VVMC_CalibratedAccX_G]
  GreaterThan4/1 -> OR1/1
  [VVMC_VehspdLo_flg] -> AND11/2, NOT4/1
  [task_time_s] -> DelayEnable/3(Ts)
  Less Than4/1 -> AND8/2
  Switch23/1 -> Switch8/3
  Constant35/1 -> GreaterThan5/2
  Constant33/1 -> Less Than3/2
  Constant20/1 -> Switch10/2
  If/4 -> If Action Subsystem3/Action
  If Action Subsystem3/1(Out1) -> Merge/4
  Asin1/1 -> Gain5/1
  [VTQD_VehActSpd_kph] -> Switch32/1
  AND5/1 -> Switch2/2
  If/3 -> If Action Subsystem2/Action
  [VVMC_CalibratedGyroYDevTs_c] -> FirstOrderFilter7/3(Ts)
  [VTQD_GearActualPosn_enum] -> Unit Delay1/1
  FirstOrderFilter7/1(out) -> Switch6/1  "VVMC_CalibratedGyroYDevAfter_Dps"
  [VTQD_VehActSpd_kph] -> Switch10/3
  MVMC_CalEstSlopeTs_Y_c/1 -> [VVMC_CalEstSlopeTs_c]  "VVMC_CalEstSlopeTs_c"
  SR_Latch2/1(latched) -> [VVMC_PitchGradeL2H_flg]  "VVMC_PitchGradeL2H_flg"
  [VVMC_CalEstSlopeTs_c] -> FirstOrderFilter5/3(Ts)
  Switch8/1 -> Unit Delay3/1, Switch2/3
  MVMC_VehspdTs_Y_c/1 -> [VVMC_VehspdTs_c]  "VVMC_VehspdTs_c"
  Switch10/1 -> MVMC_GyroYBandHi_Y_Dps/1, MVMC_GyroYBandLo_Y_Dps/1
  Constant22/1 -> DelayEnable4/2(T_delay)
  AND13/1 -> [VVMC_VehSpdHi_flg]  "VVMC_VehSpdHi_flg"
  AND12/1 -> [VVMC_Vehstop_flg]  "VVMC_Vehstop_flg"
  NOT/1 -> AND1/3  "VVMC_PitchRollingCondmet_flg"
  MVMC_GyroYBandLo_Y_Dps/1 -> [VVMC_GyroYBandLow_Dps]  "VVMC_GyroYBandLow_Dps"
  OR5/1 -> [VVMC_PitchAllcondmet_flg]  "VVMC_PitchAllcondmet_flg"
  [VVMC_RDShift_flg] -> SR_Latch6/1(set)
  [VVMC_VehspdTs_c] -> FirstOrderFilter4/3(Ts)
  Constant30/1 -> Less Than2/2
  Detect Decrease/1 -> Triggered Subsystem/Trigger
  [VVMC_VehspdLo_flg] -> NOT2/1
  [VVMC_VehSpdHi_flg] -> AND3/1
  [VVMC_VehspdLo_flg] -> NOT1/1
  NOT2/1 -> AND3/2
  [VVMC_Vehstop_flg] -> Detect Decrease/1
  SR_Latch1/1(latched) -> OR6/2  "VVMC_PitchGradeHiReset_flg"
  Detect Decrease1/1 -> Switch11/2
  OR6/1 -> [VVMC_PitchGradeReset_flg]
  [task_time_s] -> DelayEnable4/3(Ts)
  [VVMC_Vehstop_flg] -> If/3
  [VVMC_Vehstop_flg] -> Detect Decrease2/1
  Constant56/1 -> Switch5/2
  Switch11/1 -> Add2/1
  AND9/1 -> [VVMC_Vehfullstop_flg]  "VVMC_Vehfullstop_flg"
  Switch12/1 -> [VVMC_PitchIntegGradeBase_deg], Switch19/1, Unit Delay/1  "VVMC_PitchIntegGradeBase_deg"
  Unit Delay1/1 -> Equal1/1
  [VVMC_VehspdLo_flg] -> AND10/2, NOT3/1
  Detect Decrease2/1 -> Unit Delay4/1
  Equal2/1 -> AND4/1
  Constant10/1 -> Switch12/1
  [VVMC_GradeShiftDelay_flg] -> AND7/1
  [VTQD_GearActualPosn_enum] -> Equal3/1
  Constant31/1 -> Switch11/3
  Constant11/1 -> GreaterThan2/2
  Constant51/1 -> Switch31/2
  AND1/1 -> OR5/1
  NOT4/1 -> SR_Latch3/2(reset)
  [VVMC_EstPitchSlopeTs_c] -> FirstOrderFilter6/3(Ts)
  If Action Subsystem/1(Out1) -> Merge/1
  Constant13/1 -> Less Than6/2
  Constant29/1 -> Switch14/2
  Less Than6/1 -> AND9/2
  Unit Delay5/1 -> AND11/1
  Switch7/1 -> Switch13/3  "VVMC_PitchIntegGradeBaseA_deg"
  Switch14/1 -> Switch7/3
  [task_time_s] -> FirstOrderFilter7/2(Tc)
  [VVMC_CalEstSlopeTs_c] -> FirstOrderFilter3/3(Ts)
  [VTQD_GearActualPosn_enum] -> Unit Delay2/1
  [VVMC_PitchGradeL2H_flg] -> AND1/4
  Less Than3/1 -> AND8/1
  [VVMC_VehSpdHi_flg] -> Detect Decrease3/1
  Unit Delay/1 -> Add2/3
  [VVMC_PitchGradeReset_flg] -> OR7/2
  [VVMC_GradeReset_flg] -> OR5/2
  AND3/1 -> SR_Latch1/1(set)
  Less Than2/1 -> DelayEnable/1(trigger)
  Triggered Subsystem/1(Out1) -> [VVMC_BaseGrade_deg]  "VVMC_BaseGrade_deg"
  Switch6/1 -> Add2/2
  GreaterThan2/1 -> AND1/2  "VVMC_PitchVehCondmet_flg"
  [VTQD_VehActSpd_kph] -> Less Than5/1
  [VVMC_CalibratedAccX_G] -> GreaterThan/1, Less Than/1
  Switch32/1 -> MVMC_CalibratedGyroYDevTs_Y_c/1, MVMC_EstPitchSlopeTs_Y_c/1
  Unit Delay4/1 -> AND10/1
  [VVMC_Vehstop_flg] -> Detect Decrease1/1
  FirstOrderFilter6/1(out) -> [VVMC_PitchIntegGrade_deg]  "VVMC_PitchIntegGrade_deg"
  AND8/1 -> [VVMC_VehspdLo_flg]  "VVMC_VehspdLo_flg"
  SR_Latch3/1(latched) -> [VVMC_PitchGradeH2L_flg]  "VVMC_PitchGradeH2L_flg"
  NOT3/1 -> SR_Latch2/2(reset)
  Constant19/1 -> Equal3/2
  SR_Latch/1(latched) -> OR6/1  "VVMC_PitchGradeStopReset_flg"
  If/2 -> If Action Subsystem1/Action
  [VVMC_Vehstop_flg] -> AND/1
  Constant49/1 -> Less Than7/2
  Constant18/1 -> Equal1/2
  Switch25/1 -> [VVMC_PitchIntegGradeMen_deg], Unit Delay8/1  "VVMC_PitchIntegGradeMen_deg"
  OR/1 -> [VVMC_RDShift_flg]  "VVMC_RDShift_flg"
  [VVMC_PitchIntegGrade_deg] -> Switch25/3
  Unit Delay3/1 -> Switch8/1
  Constant25/1 -> Switch9/1
  Switch1/1 -> Switch23/3
  [VVMC_PitchGradeH2L_flg] -> Switch13/2
  Constant42/1 -> Switch1/2
  [task_time_s] -> FirstOrderFilter5/2(Tc)
  Add1/1 -> Asin1/1  "sum"
  FirstOrderFilter3/1(out) -> Add1/1  "VVMC_CalibratedAccXAfter_G"
  Switch31/1 -> VVMC_IMUEstSlope_Deg1/1, [VVMC_IMUEstSlope_Deg1]  "VVMC_IMUEstSlope_Deg1"
  Gain1/1 -> Add1/2  "VVMC_VehCalgAfter_G"
  [VTQD_VehActSpd_kph] -> Less Than3/1, Less Than4/1
  Switch3/1 -> FirstOrderFilter3/1(in)
  [VTQD_VehActSpd_kph] -> Switch5/1
  Constant52/1 -> Switch3/2
  [VINP_VehSpeed_kph] -> Switch5/3
  Constant14/1 -> AND5/2
  [VINP_VehSpeed_kph] -> Switch4/3
  Constant15/1 -> Switch27/2
  [VVMC_VehspdLo_flg] -> If/2
  [VINP_DIDGetDynoMode_flg] -> AND5/1
  [VINP_BrkPedalPos_pct] -> GreaterThan3/1
  Constant12/1 -> Switch6/3
  [VVMC_CalibratedGyroY_Dps] -> Switch9/3
  Less Than/1 -> AND2/2
  Constant55/1 -> Less Than/2
  Constant16/1 -> GreaterThan3/2
  Add2/1 -> Switch12/3  "VVMC_PitchIntegTotal_deg"
  Switch5/1 -> GreaterThan2/1
  Product/1 -> FirstOrderFilter7/1(in)  "VVMC_CalibratedGyroYDev_Dps"
  Equal3/1 -> AND6/1
  DelayEnable4/1(set) -> SR_Latch6/2(reset)
  Equal4/1 -> AND6/2
  [VTQD_GearActualPosn_enum] -> Equal2/1
  AND6/1 -> OR/2
  Equal1/1 -> AND4/2
  NOT1/1 -> AND/2
  Unit Delay2/1 -> Equal4/1
  [VVMC_VehspdLo_flg] -> SR_Latch/2(reset)
  Constant50/1 -> Switch30/2
  [task_time_s] -> Product/2
  AND4/1 -> OR/1
  [VVMC_HoldEstSlope_deg] -> Switch27/3
  Constant/1 -> Switch4/2
  GreaterThan/1 -> AND2/1
  [VVMC_HoldEstSlope_deg] -> Switch30/3
  Constant24/1 -> AND7/2
  Constant36/1 -> Switch28/2
  If Action Subsystem1/1(Out1) -> Merge/2
  Constant48/1 -> Switch23/2
  AND/1 -> SR_Latch/1(set)
  [VVMC_CalibratedGyroY_Dps] -> Less Than1/1
  AND2/1 -> AND1/1  "VVMC_CalibratedAccXRang_flg"
  MVMC_EstPitchSlopeTs_Y_c/1 -> [VVMC_EstPitchSlopeTs_c]  "VVMC_EstPitchSlopeTs_c"
  [VVMC_CalibratedAccX_G] -> Switch22/2
  Unit Delay8/1 -> Switch25/1
  Switch26/1 -> [VVMC_StopGrade_deg]  "VVMC_StopGrade_deg"
  Constant27/1 -> Switch16/2
  AND11/1 -> SR_Latch3/1(set)
  [VVMC_VehSpdHi_flg] -> If/1
  [VVMC_PitchGradeL2H_flg] -> Switch7/2
  [VTQD_VehActSpd_kph] -> GreaterThan5/1
  [VDHP_ActAPSPosn_pct] -> Less Than6/1
  OR7/1 -> [VVMC_GradeReset_flg]  "VVMC_GradeReset_flg"
  Switch28/1 -> Switch33/3
  [VVMC_EstSlopeCalBase_Deg] -> Switch27/1
  Detect Decrease3/1 -> Unit Delay5/1
  [VVMC_CalibratedAccX_G] -> MVMC_ACCGradeofst_Deg/2
  [VVMC_PitchIntegGrade_deg] -> If Action Subsystem1/1(In1)
  [task_time_s] -> FirstOrderFilter8/2(Tc)
  Switch13/1 -> FirstOrderFilter6/1(in)  "VVMC_PitchIntegGradeBefore_deg"
  [VINP_GRADE_deg] -> If Action Subsystem3/1(In1)
  Constant38/1 -> Less Than5/2
  Switch27/1 -> Switch11/1
  VVMC_CalibratedGyroY_Dps/1 -> [VVMC_CalibratedGyroY_Dps]
  VINP_GRADE_deg/1 -> [VINP_GRADE_deg]
  [VVMC_InitEstSlope_Deg] -> VVMC_EstSlopeCalBase_Deg/1, [VVMC_EstSlopeCalBase_Deg]  "VVMC_EstSlopeCalBase_Deg"
  VINP_LongAccel_Gps/1 -> [VINP_LongAccel_Gps]
  VINP_VehSpeed_kph/1 -> [VINP_VehSpeed_kph]
  VDHP_ActAPSPosn_pct/1 -> [VDHP_ActAPSPosn_pct]
  VTQD_GearActualPosn_enum/1 -> [VTQD_GearActualPosn_enum]
  Constant60/1 -> UnitDelay4/1
  UnitDelay4/1 -> Switch35/2
  Product4/1 -> Gain1/1
  UnitDelay3/1 -> Sum1/2
  Switch35/1 -> Product4/1
  [task_time_s] -> Product4/2
  Gain/1 -> Sum1/1, UnitDelay3/1
  Sum1/1 -> Switch35/1
  Constant8/1 -> Switch35/3
  VTQD_PreLoadPreEn_flg/1 -> [VTQD_PreLoadPreEn_flg]
  VINP_BrkPedalPos_pct/1 -> [VINP_BrkPedalPos_pct]
  VTQD_VehActSpd_kph/1 -> [VTQD_VehActSpd_kph]
  VTQD_RegenMode_enum/1 -> [VTQD_RegenMode_enum]
  VINP_DIDGetDynoMode_flg/1 -> [VINP_DIDGetDynoMode_flg]
  [VVMC_PitchAllcondmet_flg] -> Switch6/2
  VVMC_HoldEstSlope_deg/1 -> [VVMC_HoldEstSlope_deg]
  VVMC_InitEstSlope_Deg/1 -> [VVMC_InitEstSlope_Deg]
  [VVMC_CalibratedAccX_G] -> Switch3/1
  [VVMC_EstSlopeCalBase_Deg] -> Switch14/1
  [VVMC_HoldEstSlope_deg] -> Switch14/3
  [VVMC_EstSlopeCalBase_Deg] -> Switch16/1
  [VVMC_HoldEstSlope_deg] -> Switch16/3
  Constant1/1 -> Switch/2
  [VVMC_HoldEstSlope_deg] -> Switch/3
  Switch/1 -> [VVMC_VehRunSlope_deg]  "VVMC_VehRunSlope_deg"
  [VVMC_VehRunSlope_deg] -> If Action Subsystem/1(In1)
  VTQR_RrTMTqReq_Nm/1 -> [VTQR_RrTMTqReq_Nm]
  VTQR_FrTMTqReq_Nm/1 -> [VTQR_FrTMTqReq_Nm]
  VPMM_DrivetrainSelect_enum/1 -> [VPMM_DrivetrainSelect_enum]
  [VPMM_DrivetrainSelect_enum] -> Equal/1
  Constant2/1 -> Equal/2
  Equal/1 -> Switch17/2
  [VTQR_FrTMTqReq_Nm] -> Add/1
  [VTQR_RrTMTqReq_Nm] -> Add/2
  Add/1 -> Switch17/1
  [VTQR_RrTMTqReq_Nm] -> Switch18/1
  [VPMM_DrivetrainSelect_enum] -> Equal5/1
  Constant3/1 -> Equal5/2
  Equal5/1 -> Switch18/2
  Switch18/1 -> Switch17/3
  [VTQR_FrTMTqReq_Nm] -> Switch18/3
  Switch17/1 -> [VVMC_MCUTotalTq_Nm]  "VVMC_MCUTotalTq_Nm"
  Less Than5/1 -> AND12/1
  [VVMC_MCUTotalTq_Nm] -> Abs/1
  Abs/1 -> Less Than8/1
  Constant4/1 -> Less Than8/2
  Less Than8/1 -> AND12/2
  [VVMC_Vehstop_flg] -> NOT8/1
  [VVMC_VehspdLo_flg] -> NOT7/1
  GreaterThan5/1 -> AND13/1
  NOT7/1 -> AND13/2
  NOT8/1 -> AND13/3
  [VTQD_VehActSpd_kph] -> MVMC_GradeCompFlt_Y_c/1
  MVMC_GradeCompFlt_Y_c/1 -> [VVMC_GradeCompFlt_c]  "VVMC_GradeCompFlt_c"
  [VVMC_PitchIntegGradeBase_deg] -> Product1/1
  [VVMC_GradeCompFlt_c] -> Product1/2
  Product1/1 -> Add3/1
  Constant5/1 -> Subtract/1
  [VVMC_GradeCompFlt_c] -> Subtract/2
  Subtract/1 -> Product2/1
  [VVMC_HoldEstSlope_deg] -> Product2/2
  Product2/1 -> Add3/2
  Add3/1 -> [VVMC_GradeCompFlt_deg]  "VVMC_GradeCompFlt_deg"
  [VVMC_GradeCompFlt_deg] -> Switch19/3
  Switch19/1 -> Switch7/1
  Constant6/1 -> Switch19/2
  [VINP_VehSpeed_kph] -> Switch32/3
  Constant7/1 -> Switch20/2
  Switch20/1 -> Less Than2/1
  Constant23/1 -> Switch21/2
  [VINP_VehSpeed_kph] -> Switch21/3
  [VTQD_VehActSpd_kph] -> Switch21/1
  Switch21/1 -> Less Than7/1

== system vmc/VMC/VMC/MSA function/Anti-Speed Limitation ==
  VINP_HoodSW_flg : Inport
  VTQD_GearActualPosn_enum : Inport  Port=2
  VINP_SmartEcoModeSW_flg : Inport  Port=3
  VVMC_APSActive_flg : Inport  Port=4
  VVMC_IntMSACtrlSta_enum : Inport  Port=5
  AND : Logic  Inputs=3  AllPortsSameDT=off  OutDataTypeStr=boolean
  AND1 : Logic  AllPortsSameDT=off  OutDataTypeStr=boolean
  AND2 : Logic  Inputs=3  AllPortsSameDT=off  OutDataTypeStr=boolean
  AND3 : Logic  AllPortsSameDT=off  OutDataTypeStr=boolean
  AND4 : Logic  Inputs=3  AllPortsSameDT=off  OutDataTypeStr=boolean
  Constant1 : Constant  Value=KVMC_AntiSpdLimSW_flg
  Constant2 : Constant  Value=ENUM_GEARACTUALPOSN_D
  Constant3 : Constant  Value=KVMC_SmartEcoPlusSW_flg
  Constant4 : Constant  Value=ENUM_GEARACTUALPOSN_D
  Constant5 : Constant  Value=KVMC_AntiSpdLim_kph
  Constant6 : Constant  Value=KVMC_SmartEcoLimitSpd_kph
  Constant7 : Constant  Value=ENUM_ADASMSASTA_ACTIVE
  Constant8 : Constant  Value=ENUM_ADASMSASTA_ACTIVE
  Constant9 : Constant  Value=ENUM_ADASMSASTA_STANDBY
  Equal : RelationalOperator  Operator===  OutDataTypeStr=boolean  RndMeth=Simplest
  Equal1 : RelationalOperator  Operator===  OutDataTypeStr=boolean  RndMeth=Simplest
  Equal2 : RelationalOperator  Operator=~=  OutDataTypeStr=boolean  RndMeth=Simplest
  Equal3 : RelationalOperator  Operator=~=  OutDataTypeStr=boolean  RndMeth=Simplest
  Equal4 : RelationalOperator  Operator=~=  OutDataTypeStr=boolean  RndMeth=Simplest
  NOT : Logic  Operator=NOT  AllPortsSameDT=off  OutDataTypeStr=boolean
  OR : Logic  Operator=OR  AllPortsSameDT=off  OutDataTypeStr=boolean
  OR1 : Logic  Operator=OR  AllPortsSameDT=off  OutDataTypeStr=boolean
  OR2 : Logic  Operator=OR  AllPortsSameDT=off  OutDataTypeStr=boolean
  Switch : Switch  Criteria=u2 > Threshold
  VVMC_AntiSpdLimEn_flg : Outport
  VVMC_AntiLimitSpd_kph : Outport  Port=2
  VVMC_AntiSpdLimSpdEn_flg : Outport  Port=3
  VVMC_AntiSpdLimStaEn_flg : Outport  Port=4
  wires:
  [VVMC_AntiLimitSpd_kph] -> VVMC_AntiLimitSpd_kph/1
  [VVMC_AntiSpdLimSpdEn_flg] -> VVMC_AntiSpdLimSpdEn_flg/1
  [VVMC_AntiSpdLimEn_flg] -> VVMC_AntiSpdLimEn_flg/1
  [VVMC_AntiSpdLimStaEn_flg] -> VVMC_AntiSpdLimStaEn_flg/1
  [VTQD_GearActualPosn_enum] -> Equal1/1
  Constant6/1 -> Switch/3
  NOT/1 -> AND2/3
  [VTQD_GearActualPosn_enum] -> Equal/1
  Constant2/1 -> Equal/2
  Constant4/1 -> Equal1/2
  AND2/1 -> [VVMC_SmartEcoEn_flg]  "VVMC_SmartEcoEn_flg"
  Constant5/1 -> Switch/1
  [VVMC_HoodSpdLimitEn_flg] -> OR/1
  [VINP_SmartEcoModeSW_flg] -> AND1/1
  AND1/1 -> AND2/1
  Equal2/1 -> AND3/2
  Constant3/1 -> AND1/2
  Equal/1 -> AND/2
  [VVMC_AntiSpdLimEn_flg] -> AND3/1
  [VVMC_IntMSACtrlSta_enum] -> Equal4/1
  Switch/1 -> [VVMC_AntiLimitSpd_kph]  "VVMC_AntiLimitSpd_kph"
  [VVMC_IntMSACtrlSta_enum] -> Equal3/1
  AND/1 -> [VVMC_HoodSpdLimitEn_flg]  "VVMC_HoodSpdLimitEn_flg"
  Equal3/1 -> AND4/2
  Constant8/1 -> Equal3/2
  [VVMC_SmartEcoEn_flg] -> OR/2
  [VVMC_IntMSACtrlSta_enum] -> Equal2/1
  [VVMC_AntiSpdLimEn_flg] -> AND4/1
  Constant9/1 -> Equal4/2
  [VVMC_APSActive_flg] -> NOT/1
  [VVMC_HoodSpdLimitEn_flg] -> OR2/2
  Equal4/1 -> AND4/3
  Equal1/1 -> AND2/2
  AND4/1 -> OR2/1
  AND3/1 -> OR1/1
  [VVMC_HoodSpdLimitEn_flg] -> OR1/2
  Constant1/1 -> AND/3
  OR2/1 -> [VVMC_AntiSpdLimStaEn_flg]  "VVMC_AntiSpdLimStaEn_flg"
  [VVMC_HoodSpdLimitEn_flg] -> Switch/2
  OR1/1 -> [VVMC_AntiSpdLimSpdEn_flg]  "VVMC_AntiSpdLimSpdEn_flg"
  [VINP_HoodSW_flg] -> AND/1
  Constant7/1 -> Equal2/2
  OR/1 -> [VVMC_AntiSpdLimEn_flg]  "VVMC_AntiSpdLimEn_flg"
  VINP_SmartEcoModeSW_flg/1 -> [VINP_SmartEcoModeSW_flg]
  VVMC_APSActive_flg/1 -> [VVMC_APSActive_flg]
  VVMC_IntMSACtrlSta_enum/1 -> [VVMC_IntMSACtrlSta_enum]
  VTQD_GearActualPosn_enum/1 -> [VTQD_GearActualPosn_enum]
  VINP_HoodSW_flg/1 -> [VINP_HoodSW_flg]

== system vmc/VMC/VMC/MSA function/MSAActivationHandshake ==
  VTQD_SpdCtrlMode_enum : Inport
  VVMC_FeatArbitrFinal_enum : Inport  Port=2
  VTQD_ExternalTqAllow_flg : Inport  Port=3
  VVMC_MeterIndSpeed_raw32 : Inport  Port=4
  VVMC_FeatSetSpdFinal_raw32 : Inport  Port=5
  VTQD_SWC2CANCELSta_flg : Inport  Port=6
  VTQD_SWC2ResUpSta_flg : Inport  Port=7
  VTQD_SWC2SetdownSta_flg : Inport  Port=8
  VVMC_MSAOvrdAllow_flg : Inport  Port=9
  VINP_Distanceunit_flg : Inport  Port=10
  VTQD_GearActualPosn_enum : Inport  Port=11
  VVMC_VMCMSACtrlAvail_flg : Inport  Port=12
  VINP_SWCType_enum : Inport  Port=13
  VTQD_SWC1CANCELSta_flg : Inport  Port=14
  VTQD_SWC1ResUpSta_flg : Inport  Port=15
  VTQD_SWC1SetdownSta_flg : Inport  Port=16
  " 1" : Constant  Value=KTQD_MSAActiveMetSpdLoMPH_mph
  " 2" : Constant  Value=ENUM_SWCTYPE_SWC2
  " 80" : Constant  Value=KTQD_MSAActiveMetSpdLo_kph
  1 : Constant  Value=KPH2MPH
  160 : Constant  Value=KTQD_MSAActiveMetSpdHi_kph
  2 : Constant  Value=KTQD_MSAActiveMetSpdHiMPH_mph
  AND : Logic  AllPortsSameDT=off  OutDataTypeStr=boolean
  AND1 : Logic  Operator=OR  AllPortsSameDT=off  OutDataTypeStr=boolean
  Cast To Boolean : DataTypeConversion  OutDataTypeStr=boolean
  Cast To Single : DataTypeConversion  OutDataTypeStr=uint8
  Cast To Single1 : DataTypeConversion  OutDataTypeStr=boolean
  Cast To Single2 : DataTypeConversion  OutDataTypeStr=single
  Cast To Single3 : DataTypeConversion  OutDataTypeStr=single
  Chart : Stateflow chart  TreatAsAtomicUnit=on
  Constant1 : Constant  Value=KVMC_CCMSASpdWar_kph
  Constant3 : Constant  Value=ENUM_ADASMSASTA_UNLIMIT
  Constant5 : Constant  Value=ENUM_FEATARBITRSTA_MSA
  Constant6 : Constant  Value=TRUE
  Constant7 : Constant  Value=FALSE
  Constant8 : Constant  Value=ENUM_ADASMSASTA_ACTIVE
  Detect Decrease2 : simulink/Logic and Bit Operations/Detect Decrease  vinit=0.0  OutDataTypeStr=boolean
  Detect Decrease3 : simulink/Logic and Bit Operations/Detect Decrease  vinit=0.0  OutDataTypeStr=boolean
  Detect Decrease4 : simulink/Logic and Bit Operations/Detect Decrease  vinit=0.0  OutDataTypeStr=boolean
  Detect Increase : simulink/Logic and Bit Operations/Detect Increase  vinit=0.0  OutDataTypeStr=boolean
  Detect Increase1 : simulink/Logic and Bit Operations/Detect Increase  vinit=0.0  OutDataTypeStr=boolean
  Detect Increase2 : simulink/Logic and Bit Operations/Detect Increase  vinit=0.0  OutDataTypeStr=boolean
  Divide : Product  Inputs=**
  Relational Operator{,1..3} (4 alike) : RelationalOperator  Operator===  OutDataTypeStr=boolean  RndMeth=Simplest
  Switch{1..6} (6 alike) : Switch  Criteria=u2 > Threshold
  u2 > 0 : Switch  Criteria=u2 > Threshold
  VVMC_IntMSACtrlSta_enum : Outport
  VVMC_IntMSASpdWar_flg : Outport  Port=2
  VVMC_IntMSAActive_flg : Outport  Port=3
  wires:
  VTQD_SWC1CANCELSta_flg/1 -> [VTQD_SWC1CANCELSta_flg]
  VTQD_SWC1ResUpSta_flg/1 -> [VTQD_SWC1ResUpSta_flg]
  VTQD_SWC1SetdownSta_flg/1 -> [VTQD_SWC1SetdownSta_flg]
  VINP_SWCType_enum/1 -> [VINP_SWCType_enum]
  Detect Decrease4/1 -> Switch5/3
  [VTQD_SWC2ResUpSta_flg] -> Detect Increase1/1
  Relational Operator3/1 -> Switch1/2, Switch4/2, Switch5/2
  Detect Increase/1 -> Switch1/1
  [VTQD_SWC2CANCELSta_flg] -> Detect Increase/1
  [VTQD_SWC1CANCELSta_flg] -> Detect Decrease2/1
  Detect Decrease2/1 -> Switch1/3
  Detect Increase2/1 -> Switch5/1
  Detect Decrease3/1 -> Switch4/3
  [VTQD_SWC1ResUpSta_flg] -> Detect Decrease3/1
  Detect Increase1/1 -> Switch4/1
  [VTQD_SWC1SetdownSta_flg] -> Detect Decrease4/1
  " 2"/1 -> Relational Operator3/2
  [VINP_SWCType_enum] -> Relational Operator3/1
  [VTQD_SWC2SetdownSta_flg] -> Detect Increase2/1
  [VVMC_VMCMSACtrlAvail_flg] -> Chart/13(VVMC_VMCMSACtrlAvail_flg)
  VVMC_VMCMSACtrlAvail_flg/1 -> [VVMC_VMCMSACtrlAvail_flg]
  [VTQD_GearActualPosn_enum] -> Chart/12(VTQD_GearActualPosn_enum)
  VTQD_GearActualPosn_enum/1 -> [VTQD_GearActualPosn_enum]
  Cast To Single3/1 -> Chart/5(KVMC_MSAActiveMetSpdLo_kph)
  Cast To Single2/1 -> Chart/3(KVMC_MSAActiveMetSpdHi_kph)
  VINP_Distanceunit_flg/1 -> [VINP_Distanceunit_flg]
  [VINP_Distanceunit_flg] -> Switch3/2
  " 1"/1 -> Switch3/1
  " 80"/1 -> Switch3/3
  160/1 -> Switch2/3
  2/1 -> Switch2/1
  [VINP_Distanceunit_flg] -> Switch2/2
  VTQD_SWC2ResUpSta_flg/1 -> [VTQD_SWC2ResUpSta_flg]
  VTQD_SWC2SetdownSta_flg/1 -> [VTQD_SWC2SetdownSta_flg]
  Switch5/1 -> Chart/11(VVMC_DetectSWCSet_flg)  "VVMC_DetectSWCSet_flg"
  Switch4/1 -> Chart/10(VVMC_DetectSWCRes_flg)  "VVMC_DetectSWCRes_flg"
  Constant7/1 -> u2 > 0/3
  Relational Operator/1 -> AND/1
  Relational Operator1/1 -> AND1/1
  Constant6/1 -> u2 > 0/1
  [VVMC_IntMSACtrlSta_enum] -> Relational Operator1/1
  Constant5/1 -> Relational Operator/2
  [VVMC_FeatArbitrFinal_enum] -> Relational Operator/1
  AND/1 -> u2 > 0/2
  Constant8/1 -> Relational Operator1/2
  [VTQD_SpdCtrlMode_enum] -> Chart/1(VTQD_SpdCtrlMode_enum)
  VTQD_SpdCtrlMode_enum/1 -> [VTQD_SpdCtrlMode_enum]
  [VTQD_ExternalTqAllow_flg] -> Chart/2(VTQD_ExternalTqAllow_flg)
  Switch2/1 -> Cast To Single2/1
  [VVMC_MeterIndSpeed_raw32] -> Chart/4(VVMC_MeterIndSpeed_raw32)
  Switch3/1 -> Cast To Single3/1
  [VVMC_FeatSetSpdFinal_raw32] -> Chart/6(VVMC_FeatSetSpdFinal_raw32)
  Switch6/1 -> Chart/7(KVMC_CCMSASpdWar_raw32)
  Switch1/1 -> Chart/8(VVMC_DetectSWCCANCEL_flg)  "VVMC_DetectSWCCANCEL_flg"
  Chart/1(VVMC_IntMSACtrlSta_enum) -> Cast To Single/1
  Chart/2(VVMC_IntMSASpdWar_flg) -> Cast To Single1/1
  u2 > 0/1 -> Cast To Boolean/1
  [VVMC_IntMSACtrlSta_enum] -> VVMC_IntMSACtrlSta_enum/1
  [VVMC_IntMSASpdWar_flg] -> VVMC_IntMSASpdWar_flg/1
  [VVMC_IntMSAActive_flg] -> VVMC_IntMSAActive_flg/1
  VVMC_FeatArbitrFinal_enum/1 -> [VVMC_FeatArbitrFinal_enum]
  VTQD_ExternalTqAllow_flg/1 -> [VTQD_ExternalTqAllow_flg]
  VTQD_SWC2CANCELSta_flg/1 -> [VTQD_SWC2CANCELSta_flg]
  VVMC_FeatSetSpdFinal_raw32/1 -> [VVMC_FeatSetSpdFinal_raw32]
  VVMC_MeterIndSpeed_raw32/1 -> [VVMC_MeterIndSpeed_raw32]
  Cast To Single1/1 -> [VVMC_IntMSASpdWar_flg]  "VVMC_IntMSASpdWar_flg"
  Cast To Boolean/1 -> [VVMC_IntMSAActive_flg]  "VVMC_IntMSAActive_flg"
  Cast To Single/1 -> [VVMC_IntMSACtrlSta_enum]  "VVMC_IntMSACtrlSta_enum"
  VVMC_MSAOvrdAllow_flg/1 -> [VVMC_MSAOvrdAllow_flg]
  [VVMC_MSAOvrdAllow_flg] -> Chart/9(VVMC_MSAOvrdAllow_flg)
  [VVMC_IntMSACtrlSta_enum] -> Relational Operator2/1
  Constant3/1 -> Relational Operator2/2
  Relational Operator2/1 -> AND1/2
  AND1/1 -> AND/2
  1/1 -> Divide/1
  Divide/1 -> Switch6/1
  Constant1/1 -> Divide/2, Switch6/3
  [VINP_Distanceunit_flg] -> Switch6/2
